simulink model "Clik_Jinv_corrado"  (R2023b)
settings: Solver=VariableStepAuto  StartTime=0.0  StopTime=15  RelTol=1e-3
StartFcn:
  | load('rbt_corrado_new.mat')
model workspace: external: MAT-File (data not in the file)
undefined symbols (not defined in the file): DiscIntNeverNeededParam, f_s
settings Model: Creator=benit  LastModifiedBy=Savio Del Peschio
settings OptimizationCC: ReuseModelBlockBuffer=off

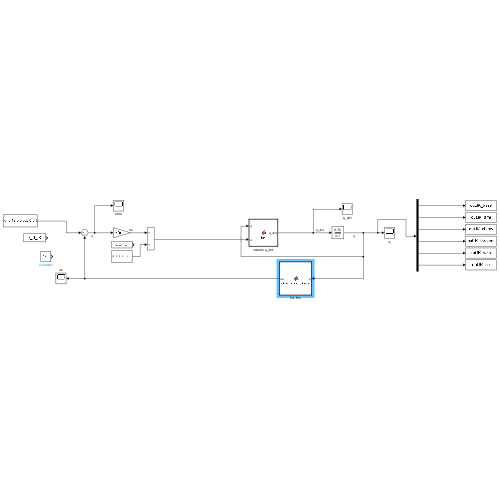
[thumbnail: Simulink's stored preview of the top-level diagram]
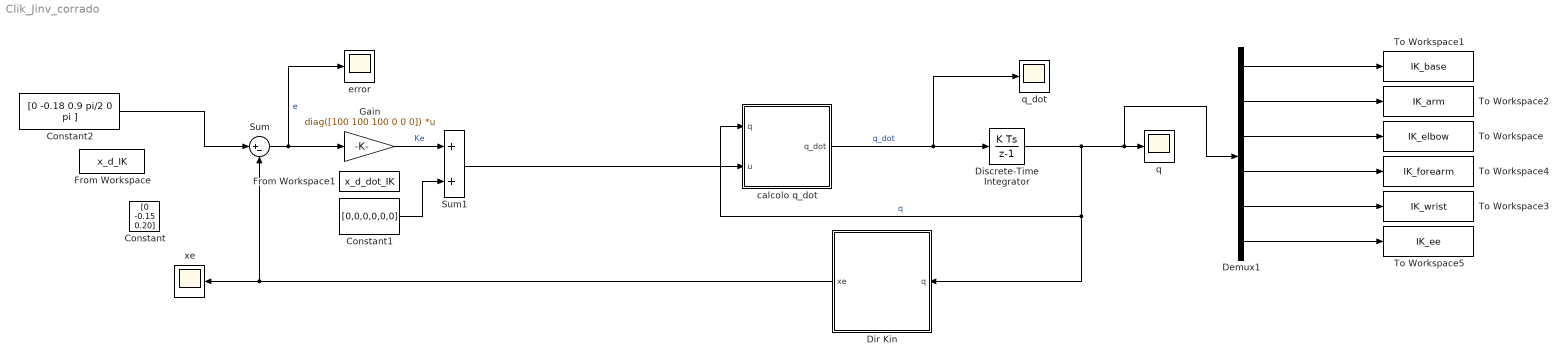
== system Clik_Jinv_corrado ==
  Constant : Constant  Value=[0 -0.15 0.20]
  Constant1 : Constant  Value=[0,0,0,0,0,0]
  Constant2 : Constant  Value=[0 -0.18 0.9 pi/2 0 pi ]
  Demux1 : Demux  Outputs=6
  Dir Kin : MATLAB Function  TreatAsAtomicUnit=on
  Discrete-Time Integrator : DiscreteIntegrator  gainval=1  InitialCondition=[0 0 0 0 0 0]'  SampleTime=1/f_s  ICPrevOutput=DiscIntNeverNeededParam  ICPrevScaledInput=DiscIntNeverNeededParam
  From Workspace : FromWorkspace  VariableName=x_d_IK
  From Workspace1 : FromWorkspace  VariableName=x_d_dot_IK
  Gain : Gain  Gain=diag([100 100 100 0 0 0])  Multiplication=Matrix(K*u)
  Sum : Sum  Inputs=|+-
  Sum1 : Sum
  To Workspace : ToWorkspace  VariableName=IK_elbow  SaveFormat=Timeseries  SampleTime=-1
  To Workspace1 : ToWorkspace  VariableName=IK_base  SaveFormat=Timeseries  SampleTime=-1
  To Workspace2 : ToWorkspace  VariableName=IK_arm  SaveFormat=Timeseries  SampleTime=-1
  To Workspace3 : ToWorkspace  VariableName=IK_wrist  SaveFormat=Timeseries  SampleTime=-1
  To Workspace4 : ToWorkspace  VariableName=IK_forearm  SaveFormat=Timeseries  SampleTime=-1
  To Workspace5 : ToWorkspace  VariableName=IK_ee  SaveFormat=Timeseries  SampleTime=-1
  calcolo q_dot : MATLAB Function  TreatAsAtomicUnit=on
  error : Scope
  q : Scope
  q_dot : Scope
  xe : Scope
  wires:
  Gain/1 -> Sum1/1  "Ke"
  Sum/1 -> error/1, Gain/1  "e"
  Discrete-Time Integrator/1 -> Dir Kin/1(q), calcolo q_dot/1(q), Demux1/1, q/1  "q"
  calcolo q_dot/1(q_dot) -> q_dot/1, Discrete-Time Integrator/1  "q_dot"
  Sum1/1 -> calcolo q_dot/2(u)
  Dir Kin/1(xe) -> xe/1, Sum/2
  Demux1/6 -> To Workspace5/1
  Demux1/2 -> To Workspace2/1
  Demux1/5 -> To Workspace3/1
  Demux1/1 -> To Workspace1/1
  Demux1/3 -> To Workspace/1
  Demux1/4 -> To Workspace4/1
  Constant2/1 -> Sum/1
  Constant1/1 -> Sum1/2

== matlab function Clik_Jinv_corrado/calcolo q_dot ==
  data: q input; u input; q_dot output
function q_dot = fcn(q, u)


theta_1 =q(1);
theta_2 =q(2);
theta_3 =q(3);
theta_4 =q(4);
theta_5 =q(5);

J = [ 
(359*cos(theta_1))/20000 + (29*sin(theta_1))/50000 - (3*cos(theta_1)*sin(theta_2))/25 - (3*cos(theta_4)*sin(theta_1))/1000 - (17*cos(theta_1)*sin(theta_2)*sin(theta_3))/100 - (19*sin(theta_1)*sin(theta_4)*sin(theta_5))/500 + (19*cos(theta_2 + theta_3)*cos(theta_1)*cos(theta_5))/500 - (3*sin(theta_2 + theta_3)*cos(theta_1)*sin(theta_4))/1000 + (17*cos(theta_1)*cos(theta_2)*cos(theta_3))/100 - (4263*cos(theta_1)*cos(theta_2)*sin(theta_3))/100000 - (4263*cos(theta_1)*cos(theta_3)*sin(theta_2))/100000 + (19*cos(theta_1)*cos(theta_2)*cos(theta_4)*sin(theta_3)*sin(theta_5))/500 + (19*cos(theta_1)*cos(theta_3)*cos(theta_4)*sin(theta_2)*sin(theta_5))/500, (359*cos(theta_1))/20000 + (29*sin(theta_1))/50000 - (3*cos(theta_1)*sin(theta_2))/25 - (3*cos(theta_4)*sin(theta_1))/1000 - (17*cos(theta_1)*sin(theta_2)*sin(theta_3))/100 - (19*sin(theta_1)*sin(theta_4)*sin(theta_5))/500 + (19*cos(theta_2 + theta_3)*cos(theta_1)*cos(theta_5))/500 - (3*sin(theta_2 + theta_3)*cos(theta_1)*sin(theta_4))/1000 + (17*cos(theta_1)*cos(theta_2)*cos(theta_3))/100 - (4263*cos(theta_1)*cos(theta_2)*sin(theta_3))/100000 - (4263*cos(theta_1)*cos(theta_3)*sin(theta_2))/100000 + (19*cos(theta_1)*cos(theta_2)*cos(theta_4)*sin(theta_3)*sin(theta_5))/500 + (19*cos(theta_1)*cos(theta_3)*cos(theta_4)*sin(theta_2)*sin(theta_5))/500,                                                                                                                                                                                          -sin(theta_1)*((4263*cos(theta_2 + theta_3))/100000 + (17*sin(theta_2 + theta_3))/100 + (3*cos(theta_2))/25 + (19*sin(theta_4 - theta_5)*cos(theta_2 + theta_3))/1000 - (19*cos(theta_2 + theta_3)*sin(theta_4 + theta_5))/1000 + (3*cos(theta_2 + theta_3)*sin(theta_4))/1000 + (19*sin(theta_2 + theta_3)*cos(theta_5))/500),                                                                                                                                                                                                                                                                  -(sin(theta_1)*(4263*cos(theta_2 + theta_3) + 17000*sin(theta_2 + theta_3) + 300*cos(theta_2 + theta_3)*sin(theta_4) + 3800*sin(theta_2 + theta_3)*cos(theta_5) - 3800*cos(theta_2 + theta_3)*cos(theta_4)*sin(theta_5)))/100000, (19*cos(theta_1)*cos(theta_4)*sin(theta_5))/500 - (3*cos(theta_1)*sin(theta_4))/1000 - (3*cos(theta_2)*cos(theta_4)*sin(theta_1)*sin(theta_3))/1000 - (3*cos(theta_3)*cos(theta_4)*sin(theta_1)*sin(theta_2))/1000 - (19*cos(theta_2)*sin(theta_1)*sin(theta_3)*sin(theta_4)*sin(theta_5))/500 - (19*cos(theta_3)*sin(theta_1)*sin(theta_2)*sin(theta_4)*sin(theta_5))/500, (19*cos(theta_1)*cos(theta_5)*sin(theta_4))/500 - (19*cos(theta_2)*cos(theta_3)*sin(theta_1)*sin(theta_5))/500 + (19*sin(theta_1)*sin(theta_2)*sin(theta_3)*sin(theta_5))/500 + (19*cos(theta_2)*cos(theta_4)*cos(theta_5)*sin(theta_1)*sin(theta_3))/500 + (19*cos(theta_3)*cos(theta_4)*cos(theta_5)*sin(theta_1)*sin(theta_2))/500;
(359*sin(theta_1))/20000 - (29*cos(theta_1))/50000 + (3*cos(theta_1)*cos(theta_4))/1000 - (3*sin(theta_1)*sin(theta_2))/25 - (4263*cos(theta_2)*sin(theta_1)*sin(theta_3))/100000 - (4263*cos(theta_3)*sin(theta_1)*sin(theta_2))/100000 + (19*cos(theta_1)*sin(theta_4)*sin(theta_5))/500 - (17*sin(theta_1)*sin(theta_2)*sin(theta_3))/100 + (19*cos(theta_2 + theta_3)*cos(theta_5)*sin(theta_1))/500 - (3*sin(theta_2 + theta_3)*sin(theta_1)*sin(theta_4))/1000 + (17*cos(theta_2)*cos(theta_3)*sin(theta_1))/100 + (19*cos(theta_2)*cos(theta_4)*sin(theta_1)*sin(theta_3)*sin(theta_5))/500 + (19*cos(theta_3)*cos(theta_4)*sin(theta_1)*sin(theta_2)*sin(theta_5))/500, (359*sin(theta_1))/20000 - (29*cos(theta_1))/50000 + (3*cos(theta_1)*cos(theta_4))/1000 - (3*sin(theta_1)*sin(theta_2))/25 - (4263*cos(theta_2)*sin(theta_1)*sin(theta_3))/100000 - (4263*cos(theta_3)*sin(theta_1)*sin(theta_2))/100000 + (19*cos(theta_1)*sin(theta_4)*sin(theta_5))/500 - (17*sin(theta_1)*sin(theta_2)*sin(theta_3))/100 + (19*cos(theta_2 + theta_3)*cos(theta_5)*sin(theta_1))/500 - (3*sin(theta_2 + theta_3)*sin(theta_1)*sin(theta_4))/1000 + (17*cos(theta_2)*cos(theta_3)*sin(theta_1))/100 + (19*cos(theta_2)*cos(theta_4)*sin(theta_1)*sin(theta_3)*sin(theta_5))/500 + (19*cos(theta_3)*cos(theta_4)*sin(theta_1)*sin(theta_2)*sin(theta_5))/500,                                                                                                                                                                                           cos(theta_1)*((4263*cos(theta_2 + theta_3))/100000 + (17*sin(theta_2 + theta_3))/100 + (3*cos(theta_2))/25 + (19*sin(theta_4 - theta_5)*cos(theta_2 + theta_3))/1000 - (19*cos(theta_2 + theta_3)*sin(theta_4 + theta_5))/1000 + (3*cos(theta_2 + theta_3)*sin(theta_4))/1000 + (19*sin(theta_2 + theta_3)*cos(theta_5))/500),                                                                                                                                                                                                                                                                   (cos(theta_1)*(4263*cos(theta_2 + theta_3) + 17000*sin(theta_2 + theta_3) + 300*cos(theta_2 + theta_3)*sin(theta_4) + 3800*sin(theta_2 + theta_3)*cos(theta_5) - 3800*cos(theta_2 + theta_3)*cos(theta_4)*sin(theta_5)))/100000, (19*cos(theta_4)*sin(theta_1)*sin(theta_5))/500 - (3*sin(theta_1)*sin(theta_4))/1000 + (3*cos(theta_1)*cos(theta_2)*cos(theta_4)*sin(theta_3))/1000 + (3*cos(theta_1)*cos(theta_3)*cos(theta_4)*sin(theta_2))/1000 + (19*cos(theta_1)*cos(theta_2)*sin(theta_3)*sin(theta_4)*sin(theta_5))/500 + (19*cos(theta_1)*cos(theta_3)*sin(theta_2)*sin(theta_4)*sin(theta_5))/500, (19*cos(theta_5)*sin(theta_1)*sin(theta_4))/500 + (19*cos(theta_1)*cos(theta_2)*cos(theta_3)*sin(theta_5))/500 - (19*cos(theta_1)*sin(theta_2)*sin(theta_3)*sin(theta_5))/500 - (19*cos(theta_1)*cos(theta_2)*cos(theta_4)*cos(theta_5)*sin(theta_3))/500 - (19*cos(theta_1)*cos(theta_3)*cos(theta_4)*cos(theta_5)*sin(theta_2))/500;
                                                                                                                                                                                                                                                                                                                                                                                                                                                                                                                                                                                                                                                                             0,                                                                                                                                                                                                                                                                                                                                                                                                                                                                                                                                                                                                                                                                              0, (17*cos(theta_2)*cos(theta_3))/100 - (3*sin(theta_2))/25 - (4263*cos(theta_2)*sin(theta_3))/100000 - (4263*cos(theta_3)*sin(theta_2))/100000 - (17*sin(theta_2)*sin(theta_3))/100 - (3*cos(theta_2)*sin(theta_3)*sin(theta_4))/1000 - (3*cos(theta_3)*sin(theta_2)*sin(theta_4))/1000 - (19*cos(theta_5)*sin(theta_2)*sin(theta_3))/500 + (19*cos(theta_2)*cos(theta_3)*cos(theta_5))/500 + (19*cos(theta_2)*cos(theta_4)*sin(theta_3)*sin(theta_5))/500 + (19*cos(theta_3)*cos(theta_4)*sin(theta_2)*sin(theta_5))/500, (17*cos(theta_2)*cos(theta_3))/100 - (4263*cos(theta_2)*sin(theta_3))/100000 - (4263*cos(theta_3)*sin(theta_2))/100000 - (17*sin(theta_2)*sin(theta_3))/100 - (3*cos(theta_2)*sin(theta_3)*sin(theta_4))/1000 - (3*cos(theta_3)*sin(theta_2)*sin(theta_4))/1000 - (19*cos(theta_5)*sin(theta_2)*sin(theta_3))/500 + (19*cos(theta_2)*cos(theta_3)*cos(theta_5))/500 + (19*cos(theta_2)*cos(theta_4)*sin(theta_3)*sin(theta_5))/500 + (19*cos(theta_3)*cos(theta_4)*sin(theta_2)*sin(theta_5))/500,                                                                                                                                                                                                                                                                                              (cos(theta_2 + theta_3)*(3*cos(theta_4) + 38*sin(theta_4)*sin(theta_5)))/1000,                                                                                                       (19*cos(theta_4)*cos(theta_5)*sin(theta_2)*sin(theta_3))/500 - (19*cos(theta_3)*sin(theta_2)*sin(theta_5))/500 - (19*cos(theta_2)*cos(theta_3)*cos(theta_4)*cos(theta_5))/500 - (19*cos(theta_2)*sin(theta_3)*sin(theta_5))/500;
                                                                                                                                                                                                                                                                                                                                                                                                                                                                                                                                                                                                                                                                             0,                                                                                                                                                                                                                                                                                                                                                                                                                                                                                                                                                                                                                                                                              0,                                                                                                                                                                                                                                                                                                                                                                                                                                                                                                           -cos(theta_1),                                                                                                                                                                                                                                                                                                                                                                                                                                                                                     -cos(theta_1),                                                                                                                                                                                                                                                                                                                                        cos(theta_2 + theta_3)*sin(theta_1),                                                                                                                                                                                                            cos(theta_1)*cos(theta_4) - sin(theta_4)*(cos(theta_2)*sin(theta_1)*sin(theta_3) + cos(theta_3)*sin(theta_1)*sin(theta_2));
                                                                                                                                                                                                                                                                                                                                                                                                                                                                                                                                                                                                                                                                             0,                                                                                                                                                                                                                                                                                                                                                                                                                                                                                                                                                                                                                                                                              0,                                                                                                                                                                                                                                                                                                                                                                                                                                                                                                           -sin(theta_1),                                                                                                                                                                                                                                                                                                                                                                                                                                                                                     -sin(theta_1),                                                                                                                                                                                                                                                                                                                                       -cos(theta_2 + theta_3)*cos(theta_1),                                                                                                                                                                                                            cos(theta_4)*sin(theta_1) + sin(theta_4)*(cos(theta_1)*cos(theta_2)*sin(theta_3) + cos(theta_1)*cos(theta_3)*sin(theta_2));
                                                                                                                                                                                                                                                                                                                                                                                                                                                                                                                                                                                                                                                                            1,                                                                                                                                                                                                                                                                                                                                                                                                                                                                                                                                                                                                                                                                              1,                                                                                                                                                                                                                                                                                                                                                                                                                                                                                                                       0,                                                                                                                                                                                                                                                                                                                                                                                                                                                                                                 0,                                                                                                                                                                                                                                                                                                                                                     sin(theta_2 + theta_3),                                                                                                                                                                                                                                                                                                   cos(theta_2 + theta_3)*sin(theta_4)];


q_dot = pinv(J)*u;

end

== matlab function Clik_Jinv_corrado/Dir Kin ==
  data: q input; xe output
function xe = cinematica_diretta(q)
 
theta_1 =q(1);
theta_2 =q(2);
theta_3 =q(3);
theta_4 =q(4);
theta_5 =q(5);
theta_6 =q(6);


Te=[cos(theta_6)*(cos(theta_1)*cos(theta_4) - sin(theta_4)*(cos(theta_2)*sin(theta_1)*sin(theta_3) + cos(theta_3)*sin(theta_1)*sin(theta_2))) - sin(theta_6)*(cos(theta_5)*(cos(theta_1)*sin(theta_4) + cos(theta_4)*(cos(theta_2)*sin(theta_1)*sin(theta_3) + cos(theta_3)*sin(theta_1)*sin(theta_2))) + sin(theta_5)*(sin(theta_1)*sin(theta_2)*sin(theta_3) - cos(theta_2)*cos(theta_3)*sin(theta_1))), - sin(theta_6)*(cos(theta_1)*cos(theta_4) - sin(theta_4)*(cos(theta_2)*sin(theta_1)*sin(theta_3) + cos(theta_3)*sin(theta_1)*sin(theta_2))) - cos(theta_6)*(cos(theta_5)*(cos(theta_1)*sin(theta_4) + cos(theta_4)*(cos(theta_2)*sin(theta_1)*sin(theta_3) + cos(theta_3)*sin(theta_1)*sin(theta_2))) + sin(theta_5)*(sin(theta_1)*sin(theta_2)*sin(theta_3) - cos(theta_2)*cos(theta_3)*sin(theta_1))), sin(theta_5)*(cos(theta_1)*sin(theta_4) + cos(theta_4)*(cos(theta_2)*sin(theta_1)*sin(theta_3) + cos(theta_3)*sin(theta_1)*sin(theta_2))) - cos(theta_5)*(sin(theta_1)*sin(theta_2)*sin(theta_3) - cos(theta_2)*cos(theta_3)*sin(theta_1)), (359*sin(theta_1))/20000 - (29*cos(theta_1))/50000 + (3*cos(theta_1)*cos(theta_4))/1000 - (3*sin(theta_1)*sin(theta_2))/25 - (4263*cos(theta_2)*sin(theta_1)*sin(theta_3))/100000 - (4263*cos(theta_3)*sin(theta_1)*sin(theta_2))/100000 + (19*cos(theta_1)*sin(theta_4)*sin(theta_5))/500 - (17*sin(theta_1)*sin(theta_2)*sin(theta_3))/100 + (19*cos(theta_2 + theta_3)*cos(theta_5)*sin(theta_1))/500 - (3*sin(theta_2 + theta_3)*sin(theta_1)*sin(theta_4))/1000 + (17*cos(theta_2)*cos(theta_3)*sin(theta_1))/100 + (19*cos(theta_2)*cos(theta_4)*sin(theta_1)*sin(theta_3)*sin(theta_5))/500 + (19*cos(theta_3)*cos(theta_4)*sin(theta_1)*sin(theta_2)*sin(theta_5))/500;
    cos(theta_6)*(cos(theta_4)*sin(theta_1) + sin(theta_4)*(cos(theta_1)*cos(theta_2)*sin(theta_3) + cos(theta_1)*cos(theta_3)*sin(theta_2))) - sin(theta_6)*(cos(theta_5)*(sin(theta_1)*sin(theta_4) - cos(theta_4)*(cos(theta_1)*cos(theta_2)*sin(theta_3) + cos(theta_1)*cos(theta_3)*sin(theta_2))) - sin(theta_5)*(cos(theta_1)*sin(theta_2)*sin(theta_3) - cos(theta_1)*cos(theta_2)*cos(theta_3))), - sin(theta_6)*(cos(theta_4)*sin(theta_1) + sin(theta_4)*(cos(theta_1)*cos(theta_2)*sin(theta_3) + cos(theta_1)*cos(theta_3)*sin(theta_2))) - cos(theta_6)*(cos(theta_5)*(sin(theta_1)*sin(theta_4) - cos(theta_4)*(cos(theta_1)*cos(theta_2)*sin(theta_3) + cos(theta_1)*cos(theta_3)*sin(theta_2))) - sin(theta_5)*(cos(theta_1)*sin(theta_2)*sin(theta_3) - cos(theta_1)*cos(theta_2)*cos(theta_3))), sin(theta_5)*(sin(theta_1)*sin(theta_4) - cos(theta_4)*(cos(theta_1)*cos(theta_2)*sin(theta_3) + cos(theta_1)*cos(theta_3)*sin(theta_2))) + cos(theta_5)*(cos(theta_1)*sin(theta_2)*sin(theta_3) - cos(theta_1)*cos(theta_2)*cos(theta_3)), (3*cos(theta_1)*sin(theta_2))/25 - (29*sin(theta_1))/50000 - (359*cos(theta_1))/20000 + (3*cos(theta_4)*sin(theta_1))/1000 + (17*cos(theta_1)*sin(theta_2)*sin(theta_3))/100 + (19*sin(theta_1)*sin(theta_4)*sin(theta_5))/500 - (19*cos(theta_2 + theta_3)*cos(theta_1)*cos(theta_5))/500 + (3*sin(theta_2 + theta_3)*cos(theta_1)*sin(theta_4))/1000 - (17*cos(theta_1)*cos(theta_2)*cos(theta_3))/100 + (4263*cos(theta_1)*cos(theta_2)*sin(theta_3))/100000 + (4263*cos(theta_1)*cos(theta_3)*sin(theta_2))/100000 - (19*cos(theta_1)*cos(theta_2)*cos(theta_4)*sin(theta_3)*sin(theta_5))/500 - (19*cos(theta_1)*cos(theta_3)*cos(theta_4)*sin(theta_2)*sin(theta_5))/500;
                                                                                                                                                                                                                                             sin(theta_6)*(sin(theta_2 + theta_3)*sin(theta_5) + cos(theta_2 + theta_3)*cos(theta_4)*cos(theta_5)) + cos(theta_2 + theta_3)*cos(theta_6)*sin(theta_4),                                                                                                                                                                                                                                                cos(theta_6)*(sin(theta_2 + theta_3)*sin(theta_5) + cos(theta_2 + theta_3)*cos(theta_4)*cos(theta_5)) - cos(theta_2 + theta_3)*sin(theta_4)*sin(theta_6),                                                                                                                                                     sin(theta_2 + theta_3)*cos(theta_5) - cos(theta_2 + theta_3)*cos(theta_4)*sin(theta_5),                                                                                                                                                                                                                                                                                                                                                  (4263*cos(theta_2 + theta_3))/100000 + (17*sin(theta_2 + theta_3))/100 + (3*cos(theta_2))/25 + (19*sin(theta_4 - theta_5)*cos(theta_2 + theta_3))/1000 - (19*cos(theta_2 + theta_3)*sin(theta_4 + theta_5))/1000 + (3*cos(theta_2 + theta_3)*sin(theta_4))/1000 + (19*sin(theta_2 + theta_3)*cos(theta_5))/500 + 11821/100000;
                                                                                                                                                                                                                                                                                                                                                                                                    0,                                                                                                                                                                                                                                                                                                                                                                                                       0,                                                                                                                                                                                                                                          0,                                                                                                                                                                                                                                                                                                                                                                                                                                                                                                                                                                                                                                                                              1;
                                                                                                                                                                                                                                                                                                                                                                                                    0,                                                                                                                                                                                                                                                                                                                                                                                                       0,                                                                                                                                                                                                                                          0,                                                                                                                                                                                                                                                                                                                                                                        1];
phy=atan2(Te(2,1),Te(1,1));
theta=atan2(-Te(3,1),sqrt(Te(3,2)^2+Te(3,3)^2));
psy=atan2(Te(3,2),Te(3,3));

xe= [Te(1:3,4);phy;theta;psy];
 
end
